simulink model "problem1"  (R2018b)
settings: Solver=ode45  StartTime=0.0  StopTime=10.0  RelTol=1e-3  EnableMultiTasking=on
undefined symbols (not defined in the file): b, g, k, m, p, z0
settings Model: Creator=xiuyang  LastModifiedBy=Yizhan
settings DataIOCC: LimitDataPoints=on  SaveFormat=Array
settings OptimizationCC: LifeSpan=inf
settings DebuggingCC: UnderspecifiedInitializationDetection=Classic  MergeDetectMultiDrivingBlocksExec=none  SolverPrmCheckMsg=warning  StateNameClashWarn=warning  SFUnexpectedBacktrackingDiag=warning  SFNoUnconditionalDefaultTransitionDiag=warning
settings HardwareCC: ProdBitPerPointer=32  ProdBitPerSizeT=32  ProdBitPerPtrDiffT=32  ProdLargestAtomicFloat=None  ProdIntDivRoundTo=Undefined  ProdEndianess=Unspecified  ProdWordSize=32  ProdHWDeviceType=32-bit Generic
settings ModelReferenceCC: PropagateSignalLabelsOutOfModel=off
settings SFSimCC: SimUseLocalCustomCode=off
settings RTWCC: RTWUseLocalCustomCode=off
settings CodeAppCC: StateflowObjectComments=on
settings GRTTargetCC: TargetLangStandard=C89/C90 (ANSI)  GeneratePreprocessorConditionals=Disable all
settings ConfigComp: CovMetricSettings=dw  CovHtmlReporting=on  CovSaveCumulativeToWorkspaceVar=on  CovSaveSingleToWorkspaceVar=on  CovExternalEMLEnable=off

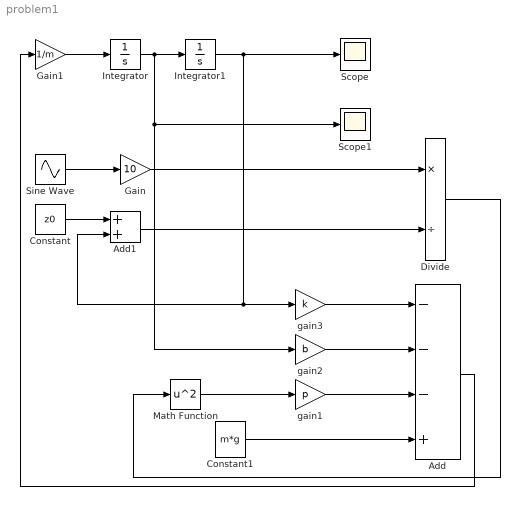
== system problem1 ==
  Add : Sum  Inputs=---+
  Add1 : Sum
  Constant : Constant  Value=z0
  Constant1 : Constant  Value=m*g
  Divide : Product  Inputs=*/
  Gain : Gain  Gain=10
  Gain1 : Gain  Gain=1/m
  Integrator : Integrator
  Integrator1 : Integrator  InitialCondition=0.1
  Math Function : Math  Operator=square  SaturateOnIntegerOverflow=on
  Scope : Scope
  Scope1 : Scope
  Sine Wave : Sin  Frequency=10  SampleTime=0
  gain1 : Gain  Gain=p
  gain2 : Gain  Gain=b
  gain3 : Gain  Gain=k
  wires:
  Integrator/1 -> Scope1/1, gain2/1, Integrator1/1
  Integrator1/1 -> gain3/1, Add1/2, Scope/1
  gain3/1 -> Add/1
  gain2/1 -> Add/2
  Divide/1 -> Math Function/1
  Math Function/1 -> gain1/1
  gain1/1 -> Add/3
  Constant/1 -> Add1/1
  Add/1 -> Gain1/1
  Sine Wave/1 -> Gain/1
  Gain/1 -> Divide/1
  Add1/1 -> Divide/2
  Constant1/1 -> Add/4
  Gain1/1 -> Integrator/1
